simulink model "ROPOD_Control_SIM"  (R2017b)
settings: Solver=VariableStepAuto  StartTime=0.0  StopTime=inf  RelTol=1e-3
values from neighbouring files (symbols this model uses):
  AgentNumber = 1    [init_model.m]
  FFtheta_intia = 0    [init_model.m]
  FFxy_mass = 0*80    (= 0)    [init_model.m]
  flock_FFtheta_friction = 50    [init_model.m]
  flock_FFxy_friction = 100    [init_model.m]
  I_fhz_ddelta_cntr = 0    [init_model.m]
  I_fhz_dtheta_cntr = 0.3    [init_model.m]
  I_fhz_dtheta_flock_cntr = 0.1    [init_model.m]
  I_fhz_dvarphi_cntr = 0    [init_model.m]
  I_fhz_dxdy_cntr = 0.25    [init_model.m]
  I_fhz_dxdy_flock_cntr = 0.1    [init_model.m]
  K_gain_ddelta_cntr = 0.1    [init_model.m]
  K_gain_dtheta_cntr = 150    [init_model.m]
  K_gain_dtheta_flock_cntr = 100    [init_model.m]
  K_gain_dvarphi_cntr = 0.05    [init_model.m]
  K_gain_dxdy_cntr = 200    [init_model.m]
  K_gain_dxdy_flock_cntr = 200    [init_model.m]
  LL_wp_fhz_ddelta_cntr = 2    [init_model.m]
  LL_wp_fhz_dtheta_cntr = 20    [init_model.m]
  LL_wp_fhz_dtheta_flock_cntr = 20    [init_model.m]
  LL_wp_fhz_dvarphi_cntr = 10    [init_model.m]
  LL_wp_fhz_dxdy_cntr = 20    [init_model.m]
  LL_wp_fhz_dxdy_flock_cntr = 20    [init_model.m]
  LL_wz_fhz_ddelta_cntr = 2    [init_model.m]
  LL_wz_fhz_dtheta_cntr = 20    [init_model.m]
  LL_wz_fhz_dtheta_flock_cntr = 20    [init_model.m]
  LL_wz_fhz_dvarphi_cntr = 2    [init_model.m]
  LL_wz_fhz_dxdy_cntr = 20    [init_model.m]
  LL_wz_fhz_dxdy_flock_cntr = 20    [init_model.m]
  LPF_fhz_ddelta_cntr = 50    [init_model.m]
  LPF_fhz_ddelta_meas = 50    [init_model.m]
  LPF_fhz_dtheta_cntr = 100    [init_model.m]
  LPF_fhz_dtheta_flock_cntr = 40    [init_model.m]
  LPF_fhz_dvarphi_cntr = 50    [init_model.m]
  LPF_fhz_dvarphi_meas = 50    [init_model.m]
  LPF_fhz_dxdy_cntr = 100    [init_model.m]
  LPF_fhz_dxdy_flock_cntr = 40    [init_model.m]
  max_flock_acc_theta = 0.5    [init_model.m]
  max_flock_acc_xy = 0.5    [init_model.m]
  max_flock_vel_theta = 1.0    (= 1)    [init_model.m]
  max_flock_vel_xy = 1.0    (= 1)    [init_model.m]
  max_hw_tau = 7.0    (= 7)    [init_model.m]
  max_ropod_acc_theta = 1.6    [init_model.m]
  max_ropod_acc_xy = 2.0    (= 2)    [init_model.m]
  max_ropod_sw_force = 500    [init_model.m]
  max_ropod_sw_tau = 250    [init_model.m]
  max_ropod_vel_theta = 1.6    [init_model.m]
  max_ropod_vel_xy = 2.0    (= 2)    [init_model.m]
  max_sw_current = 10    [init_model.m]
  Nagents = 2    [init_model.m]
  Nwheels = 4    [Jqwl_numeric_function.m]    (also in S_matrix.m; extract_kinmodel_parameters.m; init_model.m; tau_optimal_dist_vec_fun.m)
  pivot_offs_sws = [0.0243    0.4689    0.3384    5.9050]    [init_model.m]
  ropod_kinmodel_pv = struct2array(ropod_kinmodel_param)    [set_ropod_KinModparams.m]
  ropod_position_inflock = [-1 0 3.1416]    [init_model.m]
  SW_COM1_ENABLE1 = hex2dec('0001')    [init_model.m]
  SW_COM1_ENABLE2 = hex2dec('0002')    [init_model.m]
  SW_COM1_MODE_TORQUE = bitshift(hex2dec('0000'),2)    [init_model.m]
  SW_COM1_MODE_VELOCITY = bitshift(hex2dec('0002'),2)    [init_model.m]
  SW_COM1_USE_TS = hex2dec('8000')    [init_model.m]
  sw_tau_2_current = 1/motor_physical_parameters.torqueconstant.value    [init_model.m]
  Tinit = 2    [init_model.m]
  Ts = 0.001    [init_model.m]
  Ts_MPC = 0.01    [init_model.m]
  Tsflck = 0.01    [init_model.m]
undefined symbols (not defined in the file or in its folder): acc_limit, accmax, b_cx, b_cy, b_rx, bus_size, comp_enable, Desired, DiscIntNeverNeededParam, Fcgain, gdis, k_cx, k_cy, live_tuning, m_robot, Nominal, Nominal_x, Nominal_y, offsets, portwidth, sizes, types, vel_limit, vmax1, vmax2
libraries: simulink x90, cstblocks x66, dspsigops x12, dspnetwork x4
(part 3 of 8)

== system ROPOD_Control_SIM/RopodTorqueDistribution/wheel flip compensation ==
  varphi_tau_sp_in : Inport
  ropod_kin_param : Inport  Port=2
  flip_comp_factor : Inport  Port=3
  sw_conf : Inport  Port=4
  Bus Selector1 : BusSelector  OutputSignals=max_current,sw_tau_2_current
  Constant : Constant  Value=10
  Demux : Demux  Outputs=8
  Divide : Product  Inputs=*/
  MATLAB Function1 : MATLAB Function  TreatAsAtomicUnit=on
  MATLAB Function2 : MATLAB Function  TreatAsAtomicUnit=on
  MATLAB Function3 : MATLAB Function  TreatAsAtomicUnit=on
  MATLAB Function4 : MATLAB Function  TreatAsAtomicUnit=on
  Mux : Mux  Inputs=8
  Terminator{,1..3} (4 alike) : Terminator
  varphi_tau_sp_out : Outport
  wires:
  varphi_tau_sp_in/1 -> Demux/1
  ropod_kin_param/1 -> [ropod_kin_param]
  flip_comp_factor/1 -> [kmax]
  Demux/2 -> MATLAB Function4/2(tr)
  Demux/1 -> MATLAB Function4/1(tl)
  [kmax] -> MATLAB Function4/4(kmax)
  [ropod_kin_param] -> MATLAB Function4/3(ropod_kinmodel_param_vec)
  MATLAB Function4/1(tl_out) -> Mux/1
  MATLAB Function4/2(tr_out) -> Mux/2
  MATLAB Function4/3(sc) -> Terminator/1
  Mux/1 -> varphi_tau_sp_out/1
  Constant/1 -> [Fthr]
  [Fthr] -> MATLAB Function4/5(Fthr)
  Divide/1 -> [tau_max]
  [tau_max] -> MATLAB Function4/6(tau_max)
  MATLAB Function1/3(sc) -> Terminator1/1
  Demux/4 -> MATLAB Function1/2(tr)
  [Fthr] -> MATLAB Function1/5(Fthr)
  MATLAB Function1/2(tr_out) -> Mux/4
  Demux/3 -> MATLAB Function1/1(tl)
  [ropod_kin_param] -> MATLAB Function1/3(ropod_kinmodel_param_vec)
  [kmax] -> MATLAB Function1/4(kmax)
  MATLAB Function1/1(tl_out) -> Mux/3
  [tau_max] -> MATLAB Function1/6(tau_max)
  Demux/7 -> MATLAB Function3/1(tl)
  [kmax] -> MATLAB Function3/4(kmax)
  Demux/8 -> MATLAB Function3/2(tr)
  [ropod_kin_param] -> MATLAB Function2/3(ropod_kinmodel_param_vec)
  MATLAB Function3/2(tr_out) -> Mux/8
  Demux/5 -> MATLAB Function2/1(tl)
  [tau_max] -> MATLAB Function2/6(tau_max)
  [tau_max] -> MATLAB Function3/6(tau_max)
  [Fthr] -> MATLAB Function2/5(Fthr)
  MATLAB Function3/1(tl_out) -> Mux/7
  [Fthr] -> MATLAB Function3/5(Fthr)
  MATLAB Function2/3(sc) -> Terminator2/1
  MATLAB Function3/3(sc) -> Terminator3/1
  MATLAB Function2/2(tr_out) -> Mux/6
  [kmax] -> MATLAB Function2/4(kmax)
  Demux/6 -> MATLAB Function2/2(tr)
  [ropod_kin_param] -> MATLAB Function3/3(ropod_kinmodel_param_vec)
  MATLAB Function2/1(tl_out) -> Mux/5
  Bus Selector1/1 -> Divide/1  "<max_current>"
  Bus Selector1/2 -> Divide/2  "<sw_tau_2_current>"
  sw_conf/1 -> Bus Selector1/1

== system ROPOD_Control_SIM/RopodTorqueDistribution/wheel vel cntr ==
  platform_dxdy_cntr_param : Inport
  disable : Inport  Port=2
  dvarphi_sp : Inport  Port=3
  ena_w : Inport  Port=4
  dvarphi : Inport  Port=5
  Sum : Sum  Inputs=-+|
  Wheels Velocity controller : Subsystem
  varphi_tau_setp_out : Outport
  wires:
  Wheels Velocity controller/1(varphi_tau_setp) -> varphi_tau_setp_out/1
  ena_w/1 -> Wheels Velocity controller/2(ena_w)
  Sum/1 -> Wheels Velocity controller/1(dvarphi_error)
  dvarphi/1 -> Sum/1
  dvarphi_sp/1 -> Sum/2
  disable/1 -> Wheels Velocity controller/4(reset_int)
  platform_dxdy_cntr_param/1 -> Wheels Velocity controller/3(platform_dvarphi_cntr_param)

== system ROPOD_Control_SIM/RopodVelocityController/Platorm Velocity controller ==
  note: Mass Feedforward
  reset_int : Inport
  platform_dxdy_cntr_param : Inport  Port=2
  platform_dtheta_cntr_param : Inport  Port=3
  dqr_sp : Inport  Port=4
  dqr_loc : Inport  Port=5
  Demux : Demux  Outputs=3
  Demux1 : Demux  Outputs=3
  Discrete Derivative : simulink/Discrete/Discrete Derivative  gainval=1.0  ICPrevScaledInput=0.0  OutMin=[]  OutMax=[]  OutDataType=fixdt(1, 16)  OutScaling=2^-10  DoSatur=off
  G_I_LL_LPF Controller_X : Subsystem
  G_I_LL_LPF Controller_Y : Subsystem
  G_I_LL_LPF Controller_theta : Subsystem
  Gain : Gain  Gain=FFxy_mass
  Gain1 : Gain  Gain=FFxy_mass
  Gain2 : Gain  Gain=FFtheta_intia
  Mux : Mux  Inputs=3
  Mux1 : Mux  Inputs=3
  Signal Specification : SignalSpecification  Dimensions=3
  Sum : Sum  Inputs=|+-
  Sum1 : Sum  Inputs=++|
  w_platform_setp : Outport
  wires:
  Sum/1 -> Demux/1
  G_I_LL_LPF Controller_theta/1(Out) -> Mux/3
  Demux/1 -> G_I_LL_LPF Controller_X/2(In)
  Demux/2 -> G_I_LL_LPF Controller_Y/2(In)
  G_I_LL_LPF Controller_Y/1(Out) -> Mux/2
  G_I_LL_LPF Controller_X/1(Out) -> Mux/1
  Demux/3 -> G_I_LL_LPF Controller_theta/2(In)
  dqr_sp/1 -> Sum/1, Discrete Derivative/1
  dqr_loc/1 -> Sum/2
  [param_dxdy_cntr] -> G_I_LL_LPF Controller_X/1(param)
  [param_dxdy_cntr] -> G_I_LL_LPF Controller_Y/1(param)
  [param_dtheta_cntr] -> G_I_LL_LPF Controller_theta/1(param)
  reset_int/1 -> [reset_int_cntr]
  [reset_int_cntr] -> G_I_LL_LPF Controller_X/3(reset_integrator)
  [reset_int_cntr] -> G_I_LL_LPF Controller_Y/3(reset_integrator)
  platform_dxdy_cntr_param/1 -> [param_dxdy_cntr]
  platform_dtheta_cntr_param/1 -> [param_dtheta_cntr]
  [reset_int_cntr] -> G_I_LL_LPF Controller_theta/3(reset_integrator)
  Discrete Derivative/1 -> Demux1/1
  Demux1/1 -> Gain/1
  Gain/1 -> Mux1/1
  Demux1/2 -> Gain1/1
  Gain1/1 -> Mux1/2
  Demux1/3 -> Gain2/1
  Gain2/1 -> Mux1/3
  Sum1/1 -> Signal Specification/1
  Mux1/1 -> Sum1/1
  Mux/1 -> Sum1/2
  Signal Specification/1 -> w_platform_setp/1

== system ROPOD_Control_SIM/RopodVelocityController/Subscriber vel commands1 ==
  note: set 0 for testing
  note: if no vel commands are received after 0.5 sec, stop
  base_conf : Inport
  new_cmd : Inport  Port=2
  dq_setp : Inport  Port=3
  Bus Selector1 : BusSelector  OutputSignals=max_acc_xy,max_vel_xy
  Bus Selector2 : BusSelector  OutputSignals=max_acc_xy,max_vel_xy
  Bus Selector3 : BusSelector  OutputSignals=max_acc_theta,max_vel_theta
  Compare To Constant : simulink/Logic and Bit Operations/Compare To Constant  relop=>=  const=0.5  OutDataTypeStr=boolean
  Constant : Constant  Value=0  SampleTime=Ts
  Constant1 : Constant  Value=0
  Constant2 : Constant  Value=0
  Demux : Demux  Outputs=3
  Digital Clock : DigitalClock  SampleTime=Ts
  Enabled Delay : Delay  DelayLength=1  ShowEnablePort=on  SampleTime=Ts
      settings: InputPortMap=u0,e6
  Gain{,1..5} (6 alike) : Gain  Gain=-1
  Gain6 : Gain
  Mux : Mux  Inputs=3
  Rate Limiter Dynamic : simulink/Discontinuities/Rate Limiter Dynamic
      settings: SourceProductName=Simulink
  Rate Limiter Dynamic1 : simulink/Discontinuities/Rate Limiter Dynamic
      settings: SourceProductName=Simulink
  Rate Limiter Dynamic2 : simulink/Discontinuities/Rate Limiter Dynamic
      settings: SourceProductName=Simulink
  Saturation Dynamic : simulink/Discontinuities/Saturation Dynamic  OutMin=[]  OutMax=[]  OutDataTypeStr=Inherit: Same as second input  OutDataType=fixdt(1, 16)  OutScaling=2^-10  DoSatur=off
  Saturation Dynamic1 : simulink/Discontinuities/Saturation Dynamic  OutMin=[]  OutMax=[]  OutDataTypeStr=Inherit: Same as second input  OutDataType=fixdt(1, 16)  OutScaling=2^-10  DoSatur=off
  Saturation Dynamic2 : simulink/Discontinuities/Saturation Dynamic  OutMin=[]  OutMax=[]  OutDataTypeStr=Inherit: Same as second input  OutDataType=fixdt(1, 16)  OutScaling=2^-10  DoSatur=off
  Subtract : Sum  Inputs=+-
  Switch : Switch  Criteria=u2 > Threshold
  Switch1 : Switch  Criteria=u2 > Threshold
  Switch2 : Switch  Criteria=u2 > Threshold
  dq_loc_sp : Outport
  wires:
  Demux/1 -> Switch/3
  dq_setp/1 -> Demux/1
  new_cmd/1 -> Enabled Delay/2
  Digital Clock/1 -> Enabled Delay/1, Subtract/1
  Enabled Delay/1 -> Subtract/2
  Subtract/1 -> Compare To Constant/1
  Constant/1 -> Switch/1
  Gain/1 -> Rate Limiter Dynamic/3
  Switch/1 -> Saturation Dynamic/2
  Gain1/1 -> Saturation Dynamic/3
  Saturation Dynamic/1 -> Rate Limiter Dynamic/2
  Switch1/1 -> Saturation Dynamic1/2
  Gain3/1 -> Saturation Dynamic1/3
  Constant1/1 -> Switch1/1
  Demux/2 -> Switch1/3
  Gain2/1 -> Rate Limiter Dynamic1/3
  Saturation Dynamic1/1 -> Rate Limiter Dynamic1/2
  Bus Selector2/1 -> Rate Limiter Dynamic1/1, Gain2/1  "<max_acc_xy>"
  Bus Selector2/2 -> Saturation Dynamic1/1, Gain3/1  "<max_vel_xy>"
  Bus Selector3/1 -> Rate Limiter Dynamic2/1, Gain4/1  "<max_acc_theta>"
  Saturation Dynamic2/1 -> Rate Limiter Dynamic2/2
  base_conf/1 -> Bus Selector3/1, Bus Selector2/1, Bus Selector1/1
  Switch2/1 -> Saturation Dynamic2/2
  Constant2/1 -> Switch2/1
  Demux/3 -> Switch2/3
  Gain5/1 -> Saturation Dynamic2/3
  Gain4/1 -> Rate Limiter Dynamic2/3
  Compare To Constant/1 -> Gain6/1
  Bus Selector3/2 -> Saturation Dynamic2/1, Gain5/1  "<max_vel_theta>"
  Mux/1 -> dq_loc_sp/1
  Rate Limiter Dynamic/1 -> Mux/1
  Rate Limiter Dynamic1/1 -> Mux/2
  Rate Limiter Dynamic2/1 -> Mux/3
  Bus Selector1/2 -> Saturation Dynamic/1, Gain1/1  "<max_vel_xy>"
  Bus Selector1/1 -> Rate Limiter Dynamic/1, Gain/1  "<max_acc_xy>"
  Gain6/1 -> Switch2/2, Switch1/2, Switch/2

== system ROPOD_Control_SIM/Subsystem/Ropod kinematic parameters ==
  ropod_kinmodel_pv : Constant  Value=ropod_kinmodel_pv
  ropod_kin_param : Outport
  wires:
  ropod_kinmodel_pv/1 -> ropod_kin_param/1

== system ROPOD_Control_SIM/Subsystem/Smart wheels conf1 ==
  Bus Creator : BusCreator  Inputs=9
  LPF_fhz_ddelta_meas : Constant  Value=LPF_fhz_ddelta_meas
  LPF_fhz_dvarphi_meas : Constant  Value=LPF_fhz_dvarphi_meas
  enable : Constant
  max_current : Constant  Value=max_sw_current
  pivot_offset_sw1 : Constant  Value=pivot_offs_sws(1)
  pivot_offset_sw2 : Constant  Value=pivot_offs_sws(2)
  pivot_offset_sw3 : Constant  Value=pivot_offs_sws(3)
  pivot_offset_sw4 : Constant  Value=pivot_offs_sws(4)
  sw_tau_2_current : Constant  Value=sw_tau_2_current
  sw_conf : Outport
  wires:
  enable/1 -> Bus Creator/1  "enable"
  max_current/1 -> Bus Creator/2  "max_current"
  pivot_offset_sw1/1 -> Bus Creator/4  "pivot_offs_sw1"
  pivot_offset_sw2/1 -> Bus Creator/5  "pivot_offs_sw2"
  pivot_offset_sw3/1 -> Bus Creator/6  "pivot_offs_sw3"
  pivot_offset_sw4/1 -> Bus Creator/7  "pivot_offs_sw4"
  LPF_fhz_dvarphi_meas/1 -> Bus Creator/8  "dvarphi_LPF_fhz"
  LPF_fhz_ddelta_meas/1 -> Bus Creator/9  "ddelta_LPF_fhz"
  Bus Creator/1 -> sw_conf/1
  sw_tau_2_current/1 -> Bus Creator/3  "sw_tau_2_current"

== system ROPOD_Control_SIM/Subsystem1/Compliant control ==
  Forces : Inport
  states : Inport  Port=2
  motion tuning bus : Inport  Port=3
  Demux : Demux  Outputs=3
  Gain : Gain  Gain=comp_enable
  Gain4 : Gain  Gain=Fcgain
  Ground [3,1] : Subsystem
  Ground [3,1]1 : Subsystem
  Ground [3,1]2 : Subsystem
  Impedance : Subsystem
  Manual Switch : ManualSwitch  CurrentSetting=0
  Force_out : Outport
  wires:
  Manual Switch/1 -> Gain/1
  Forces/1 -> Impedance/7(Fext), Gain4/1
  Impedance/1(Imp_force) -> Manual Switch/2
  Gain4/1 -> Manual Switch/1
  states/1 -> Demux/1
  Demux/2 -> Impedance/5(y)
  Demux/1 -> Impedance/4(x)
  Demux/3 -> Impedance/6(theta)
  Gain/1 -> Force_out/1
  motion tuning bus/1 -> Impedance/8(motion tuning bus)
  Ground [3,1]/1(Out1) -> Impedance/1(X0)
  Ground [3,1]1/1(Out1) -> Impedance/2(Y0)
  Ground [3,1]2/1(Out1) -> Impedance/3(theta0i)

== system ROPOD_Control_SIM/Subsystem1/Observer ==
  Input_force : Inport
  states : Inport  Port=2
  DOB3 : Subsystem
  DOB_x : Subsystem  Commented=on
  DOB_y : Subsystem  Commented=on
  Demux1 : Demux  Outputs=3
  To Workspace2 : ToWorkspace  VariableName=est_dist  SampleTime=-1
  Force_obs : Outport
  wires:
  Input_force/1 -> DOB3/1(Control input)
  DOB3/1(Estimated disturbance) -> Force_obs/1, To Workspace2/1
  states/1 -> Demux1/1
  Demux1/1 -> DOB3/2(x)
  Demux1/2 -> DOB3/3(y)
  Demux1/3 -> DOB3/4(theta)

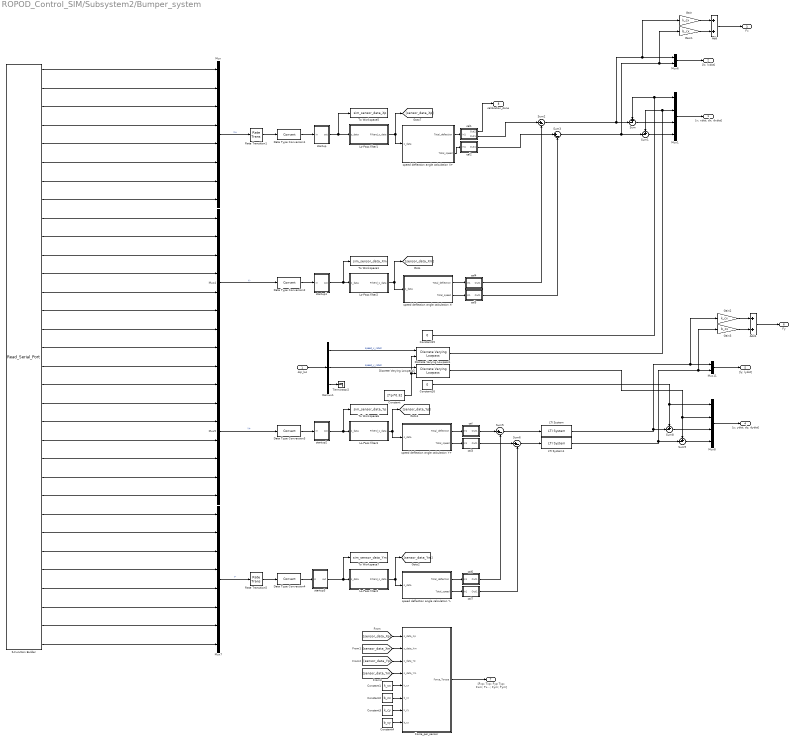
== system ROPOD_Control_SIM/Subsystem2/Bumper_system ==
  dqr_loc : Inport
  Add : Sum
  Add1 : Sum
  Constant : Constant  Value=2*pi*0.32
  Constant1 : Constant  Value=k_cx
  Constant15 : Constant  Value=0
  Constant16 : Constant  Value=0
  Constant2 : Constant  Value=b_cx
  Constant3 : Constant  Value=k_cy
  Constant4 : Constant  Value=b_cy
  Data Type Conversion{1..4} (4 alike) : DataTypeConversion
  Demux1 : Demux  Outputs=3
  Discrete Varying Lowpass1 : cstblocks/Linear Parameter Varying/Discrete Varying Lowpass  N=1  w0=0  Ts=Ts_MPC
      settings: SourceProductName=Control System Toolbox  SourceProductBaseCode=CT
  Discrete Varying Lowpass3 : cstblocks/Linear Parameter Varying/Discrete Varying Lowpass  N=1  w0=0  Ts=Ts_MPC
      settings: SourceProductName=Control System Toolbox  SourceProductBaseCode=CT
  Force_per_sensor : MATLAB Function  TreatAsAtomicUnit=on
  Gain : Gain  Gain=k_cx
  Gain1 : Gain  Gain=b_cx
  Gain2 : Gain  Gain=k_cx
  Gain3 : Gain  Gain=b_cx
  LTI System : cstblocks/LTI System  sys=hpfD_Bumper  IC=[]
  LTI System1 : cstblocks/LTI System  sys=hpfD_Bumper  IC=[]
  Lo-Pass filter1 : Subsystem
  Lo-Pass filter2 : Subsystem
  Lo-Pass filter3 : Subsystem
  Lo-Pass filter4 : Subsystem
  Mux{,4..5,7} (4 alike) : Mux  Inputs=8
  Mux1 : Mux
  Mux11 : Mux  Inputs=2
  Mux6 : Mux  Inputs=2
  Mux8 : Mux
  Rate Transition1 : RateTransition  OutPortSampleTime=Ts_MPC
  Rate Transition5 : RateTransition  OutPortSampleTime=Ts_MPC
  S-Function Builder : S-Function  InitFcn=try, set_param(gcb,'FunctionName','Read_Serial_Port'), end  FunctionName=Read_Serial_Port  SFunctionModules=Read_Serial_Port_wrapper  SFunctionDeploymentMode=off  EnableBusSupport=off  mask(S-Function Builder){}
      mask help: Simulink:masks:SFunctionBuilder_MD
      mask init:
      | val = [[.9  0.75 0.75 1 1 .9 .9 1]',[1 1 0.75 0.75 .9 .9 1 .9]'];try , sys = get_param(gcb,'SfunBuilderFcnName');if isempty(sys), sys = get_param(gcb,'FunctionName'); end,catch, sys = get_param(gcb,'FunctionName'); end
      settings: CopyFcn=set_param(gcbh,'LinkStatus','none')  PreSaveFcn=try, set_param(gcb,'FunctionName','Read_Serial_Port'), end  OpenFcn=sfunctionwizard(gcbh)
      mask Display: plot(val(:,1),val(:,2)),disp(sys), port_label('output',1,'dxp1'), port_label('output',2,'dxp2'), port_label('output',3,'dxp3'), port_label('output',4,'dxp4'), port_label('output',5,'sxp1'), port_label('output',6,'sxp2'), port_label('output',7,'sxp3'), port_label('output',8,'sxp4'), port_label('output',9,'dxm1'), port_label('output',10,'dxm2'), port_label('output',11,'dxm3'), port_label('output',12,'dxm4'), port_label('output',13,'sxm1'), port_label('output',14,'sxm2'), port_label('output',15,'sxm3'), port_label('output',16,'sxm4'), port_label('output',17,'dyp1'), port_label('output',18,'dyp2'), port_label('output',19,'dyp3'), port_label('output',20,'dyp4'), port_label('output',21,'syp1'), port_label('output',22,'syp2'), port_label('output',23,'syp3'), port_label('output',24,'syp4'), port_label('output',25,'dym1'), port_label('output',26,'dym2'), port_label('output',27,'dym3'), port_label('output',28,'dym4'), port_label('output',29,'sym1'), port_label('output',30,'sym2'), port_label('output',31,'sym3'), port_label('output',32,'sym4')
  Sum{,1,8..9} (4 alike) : Sum  Inputs=+-|
  Sum{2..3,5..6} (4 alike) : Sum  Inputs=|+-
  Terminator2 : Terminator
  To Workspace1 : ToWorkspace  VariableName=sim_sensor_data_Xm  SampleTime=-1
      settings: Save2DSignal=2-D array (concatenate along first dimension)
  To Workspace5 : ToWorkspace  VariableName=sim_sensor_data_Xp  SampleTime=-1
      settings: Save2DSignal=2-D array (concatenate along first dimension)
  To Workspace6 : ToWorkspace  VariableName=sim_sensor_data_Yp  SampleTime=-1
      settings: Save2DSignal=2-D array (concatenate along first dimension)
  To Workspace7 : ToWorkspace  VariableName=sim_sensor_data_Ym  SampleTime=-1
      settings: Save2DSignal=2-D array (concatenate along first dimension)
  cal : Subsystem
  cal1 : Subsystem
  cal2 : Subsystem
  cal3 : Subsystem
  cal4 : Subsystem
  cal5 : Subsystem
  cal6 : Subsystem
  cal7 : Subsystem
  speed deflection angle calculation X+ : MATLAB Function  TreatAsAtomicUnit=on
  speed deflection angle calculation X- : MATLAB Function  TreatAsAtomicUnit=on
  speed deflection angle calculation Y+ : MATLAB Function  TreatAsAtomicUnit=on
  speed deflection angle calculation Y- : MATLAB Function  TreatAsAtomicUnit=on
  startup : Subsystem
  startup1 : Subsystem
  startup2 : Subsystem
  startup3 : Subsystem
  "[x; xdot; dx; dxdot]" : Outport
  "[lx; lxdot]" : Outport  Port=2
  Fx : Outport  Port=3
  "[y; ydot; dy; dydot]" : Outport  Port=4
  "[ly; lydot]" : Outport  Port=5
  Fy : Outport  Port=6
  "[Fxp; Txp; Fyp Typ; Fxm; Txm; Fym; Tym] " : Outport  Port=7
  calibration_done : Outport  Port=8
  wires:
  Mux6/1 -> "[lx; lxdot]"/1
  Mux1/1 -> "[x; xdot; dx; dxdot]"/1
  Sum/1 -> Mux1/3
  Constant15/1 -> Mux1/1, Sum/1
  Sum1/1 -> Mux1/4
  Demux1/3 -> Terminator2/1
  Demux1/1 -> Discrete Varying Lowpass1/1  "speed_x_robot"
  dqr_loc/1 -> Demux1/1
  Demux1/2 -> Discrete Varying Lowpass3/1  "speed_y_robot"
  Mux/1 -> Rate Transition1/1  "X+"
  Lo-Pass filter1/1(Filterd_s_data) -> [sensor_data_Xp], speed deflection angle calculation X+/1(s_data)
  Data Type Conversion1/1 -> startup/1(in)
  Rate Transition1/1 -> Data Type Conversion1/1
  Data Type Conversion2/1 -> startup1/1(in)
  Mux4/1 -> Data Type Conversion2/1  "X-"
  Data Type Conversion3/1 -> startup2/1(in)
  Lo-Pass filter3/1(Filterd_s_data) -> speed deflection angle calculation Y+/1(s_data), [sensor_data_Yp]
  Rate Transition5/1 -> Data Type Conversion4/1
  Data Type Conversion4/1 -> startup3/1(in)
  Lo-Pass filter4/1(Filterd_s_data) -> speed deflection angle calculation Y-/1(s_data), [sensor_data_Ym]
  Mux7/1 -> Rate Transition5/1  "Y-"
  Mux5/1 -> Data Type Conversion3/1  "Y+"
  speed deflection angle calculation X+/1(Total_deflection) -> cal1/1(In1)
  cal4/1(Out1) -> Sum2/2
  cal5/1(Out1) -> Sum3/2
  speed deflection angle calculation Y-/1(Total_deflection) -> cal6/1(In1)
  speed deflection angle calculation Y+/2(Total_speed) -> cal3/1(In1)
  speed deflection angle calculation Y-/2(Total_speed) -> cal7/1(In1)
  Sum8/1 -> Mux8/3
  Mux8/1 -> "[y; ydot; dy; dydot]"/1
  Constant16/1 -> Mux8/1, Sum8/1
  Mux11/1 -> "[ly; lydot]"/1
  Sum9/1 -> Mux8/4
  Discrete Varying Lowpass3/1 -> Mux8/2, Sum9/1
  Sum5/1 -> LTI System/1
  Sum2/1 -> Sum/2, Gain/1, Mux6/1
  Sum3/1 -> Sum1/2, Gain1/1, Mux6/2
  Sum6/1 -> LTI System1/1
  startup/1(out) -> To Workspace5/1, Lo-Pass filter1/1(s_data)
  startup1/1(out) -> Lo-Pass filter2/1(s_data), To Workspace1/1
  startup2/1(out) -> Lo-Pass filter3/1(s_data), To Workspace6/1
  startup3/1(out) -> Lo-Pass filter4/1(s_data), To Workspace7/1
  Constant/1 -> Discrete Varying Lowpass3/2, Discrete Varying Lowpass1/2
  S-Function Builder/26 -> Mux7/2
  S-Function Builder/31 -> Mux7/7
  S-Function Builder/20 -> Mux5/4
  S-Function Builder/18 -> Mux5/2
  S-Function Builder/25 -> Mux7/1
  S-Function Builder/13 -> Mux4/5
  S-Function Builder/23 -> Mux5/7
  S-Function Builder/15 -> Mux4/7
  S-Function Builder/22 -> Mux5/6
  S-Function Builder/14 -> Mux4/6
  S-Function Builder/17 -> Mux5/1
  S-Function Builder/32 -> Mux7/8
  S-Function Builder/7 -> Mux/7
  S-Function Builder/19 -> Mux5/3
  S-Function Builder/21 -> Mux5/5
  S-Function Builder/8 -> Mux/8
  S-Function Builder/5 -> Mux/5
  S-Function Builder/4 -> Mux/4
  S-Function Builder/29 -> Mux7/5
  S-Function Builder/6 -> Mux/6
  S-Function Builder/1 -> Mux/1
  S-Function Builder/3 -> Mux/3
  S-Function Builder/10 -> Mux4/2
  S-Function Builder/11 -> Mux4/3
  S-Function Builder/12 -> Mux4/4
  S-Function Builder/16 -> Mux4/8
  S-Function Builder/28 -> Mux7/4
  S-Function Builder/27 -> Mux7/3
  S-Function Builder/9 -> Mux4/1
  S-Function Builder/30 -> Mux7/6
  S-Function Builder/2 -> Mux/2
  S-Function Builder/24 -> Mux5/8
  [sensor_data_Xp] -> Force_per_sensor/1(s_data_Xp)
  [sensor_data_Xm] -> Force_per_sensor/2(s_data_Xm)
  [sensor_data_Yp] -> Force_per_sensor/3(s_data_Yp)
  [sensor_data_Ym] -> Force_per_sensor/4(s_data_Ym)
  Force_per_sensor/1(Force_Torque) -> "[Fxp; Txp; Fyp Typ; Fxm; Txm; Fym; Tym] "/1
  Constant1/1 -> Force_per_sensor/5(k_cx)
  Constant2/1 -> Force_per_sensor/6(b_cx)
  Constant3/1 -> Force_per_sensor/7(k_cy)
  Constant4/1 -> Force_per_sensor/8(b_cy)
  speed deflection angle calculation X+/2(Total_speed) -> cal2/1(In1)
  speed deflection angle calculation X-/1(Total_deflection) -> cal4/1(In1)
  speed deflection angle calculation X-/2(Total_speed) -> cal5/1(In1)
  speed deflection angle calculation Y+/1(Total_deflection) -> cal/1(In1)
  cal/1(Out1) -> Sum5/1
  cal3/1(Out1) -> Sum6/1
  cal6/1(Out1) -> Sum5/2
  cal7/1(Out1) -> Sum6/2
  cal1/2(Out1) -> Sum2/1
  cal2/1(Out1) -> Sum3/1
  Lo-Pass filter2/1(Filterd_s_data) -> speed deflection angle calculation X-/1(s_data), [sensor_data_Xm]
  Discrete Varying Lowpass1/1 -> Sum1/1, Mux1/2
  cal1/1(Out2) -> calibration_done/1
  Gain/1 -> Add/1
  Gain1/1 -> Add/2
  Add/1 -> Fx/1
  Gain2/1 -> Add1/1
  LTI System1/1 -> Sum9/2, Gain3/1, Mux11/2
  Add1/1 -> Fy/1
  LTI System/1 -> Sum8/2, Gain2/1, Mux11/1
  Gain3/1 -> Add1/2

== system ROPOD_Control_SIM/Subsystem2/ZMPC_1d_x ==
  update_parameters : Inport
  "[x; xdot; d; ddot]" : Inport  Port=2
  Fd_max : Inport  Port=3
  Fd_min : Inport  Port=4
  l_max : Inport  Port=5
  l_min : Inport  Port=6
  Fr_max : Inport  Port=7
  Fr_min : Inport  Port=8
  m_r : Inport  Port=9
  b_r : Inport  Port=10
  b_c : Inport  Port=11
  k_c : Inport  Port=12
  Ts_MPC : Inport  Port=13
  Enable : EnablePort  StatesWhenEnabling=reset
  MATLAB Function : MATLAB Function  TreatAsAtomicUnit=on
  Zone MPC : MATLAB Function  TreatAsAtomicUnit=on  SystemSampleTime=Ts_MPC
  epsilon : Outport  OutputWhenDisabled=reset  InitialOutput=0
  Fx : Outport  Port=2  OutputWhenDisabled=reset  InitialOutput=0
  Feasability : Outport  Port=3  OutputWhenDisabled=reset  InitialOutput=0
  wires:
  Zone MPC/3(exitflag) -> Feasability/1
  "[x; xdot; d; ddot]"/1 -> Zone MPC/1(xk)
  Zone MPC/1(epsilon) -> epsilon/1
  Zone MPC/2(u_mpc) -> Fx/1
  m_r/1 -> MATLAB Function/1(m_r)
  b_r/1 -> MATLAB Function/2(b_r)
  b_c/1 -> MATLAB Function/3(b_c)
  k_c/1 -> MATLAB Function/4(k_c)
  Fd_max/1 -> MATLAB Function/5(Fd_max)
  Fd_min/1 -> MATLAB Function/6(Fd_min)
  Fr_max/1 -> MATLAB Function/9(Fr_max)
  Fr_min/1 -> MATLAB Function/10(Fr_min)
  Ts_MPC/1 -> MATLAB Function/11(Ts_MPC)
  update_parameters/1 -> MATLAB Function/12(update)
  MATLAB Function/1(F) -> Zone MPC/2(F)
  MATLAB Function/2(W) -> Zone MPC/3(W)
  MATLAB Function/3(c) -> Zone MPC/4(c)
  MATLAB Function/4(H) -> Zone MPC/5(H)
  MATLAB Function/5(A) -> Zone MPC/6(A)
  MATLAB Function/6(rho) -> Zone MPC/7(rho)
  l_max/1 -> MATLAB Function/7(l_max)
  l_min/1 -> MATLAB Function/8(l_min)

== system ROPOD_Control_SIM/Subsystem2/ZMPC_1d_y ==
  update_parameters : Inport
  "[x; xdot; d; ddot]" : Inport  Port=2
  Fd_max : Inport  Port=3
  Fd_min : Inport  Port=4
  l_max : Inport  Port=5
  l_min : Inport  Port=6
  Fr_max : Inport  Port=7
  Fr_min : Inport  Port=8
  m_r : Inport  Port=9
  b_r : Inport  Port=10
  b_c : Inport  Port=11
  k_c : Inport  Port=12
  Ts_MPC : Inport  Port=13
  Enable : EnablePort  StatesWhenEnabling=reset
  MATLAB Function : MATLAB Function  TreatAsAtomicUnit=on
  Zone MPC : MATLAB Function  TreatAsAtomicUnit=on  SystemSampleTime=Ts_MPC
  epsilon : Outport  OutputWhenDisabled=reset  InitialOutput=0
  Fx : Outport  Port=2  OutputWhenDisabled=reset  InitialOutput=0
  Feasability : Outport  Port=3  OutputWhenDisabled=reset  InitialOutput=0
  wires:
  Zone MPC/3(exitflag) -> Feasability/1
  "[x; xdot; d; ddot]"/1 -> Zone MPC/1(xk)
  Zone MPC/1(epsilon) -> epsilon/1
  Zone MPC/2(u_mpc) -> Fx/1
  m_r/1 -> MATLAB Function/1(m_r)
  b_r/1 -> MATLAB Function/2(b_r)
  b_c/1 -> MATLAB Function/3(b_c)
  k_c/1 -> MATLAB Function/4(k_c)
  Fd_max/1 -> MATLAB Function/5(Fd_max)
  Fd_min/1 -> MATLAB Function/6(Fd_min)
  Fr_max/1 -> MATLAB Function/9(Fr_max)
  Fr_min/1 -> MATLAB Function/10(Fr_min)
  Ts_MPC/1 -> MATLAB Function/11(Ts_MPC)
  update_parameters/1 -> MATLAB Function/12(update)
  MATLAB Function/1(F) -> Zone MPC/2(F)
  MATLAB Function/2(W) -> Zone MPC/3(W)
  MATLAB Function/3(c) -> Zone MPC/4(c)
  MATLAB Function/4(H) -> Zone MPC/5(H)
  MATLAB Function/5(A) -> Zone MPC/6(A)
  MATLAB Function/6(rho) -> Zone MPC/7(rho)
  l_max/1 -> MATLAB Function/7(l_max)
  l_min/1 -> MATLAB Function/8(l_min)

== system ROPOD_Control_SIM/FlockController/Flock Velocity controller/G_I_LL_LPF Controller_flock_Theta ==
  param : Inport
  In : Inport  Port=2
  reset_integrator : Inport  Port=3
  Bus Selector : BusSelector  OutputSignals=P_gain,I_freq_hz,LL_zero_fhz,LL_pole_fhz,LPF_fhz
  Discrete Varying Lowpass3 : cstblocks/Linear Parameter Varying/Discrete Varying Lowpass  N=1  w0=0  Ts=Tsflck
      settings: SourceProductName=Control System Toolbox  SourceProductBaseCode=CT
  Gain2 : Gain  Gain=2*pi
  Product5 : Product
  Shapeit Integrator (Tustin) : Subsystem
  Shapeit Lead-Lag (Tustin) : Subsystem
  Out : Outport
  wires:
  Gain2/1 -> Discrete Varying Lowpass3/2
  Product5/1 -> Shapeit Integrator (Tustin)/1(In)
  Discrete Varying Lowpass3/1 -> Out/1
  Shapeit Integrator (Tustin)/1(Out) -> Shapeit Lead-Lag (Tustin)/1(In)
  Bus Selector/1 -> Product5/2  "<P_gain>"
  Bus Selector/2 -> Shapeit Integrator (Tustin)/2(I_fhz)  "<I_freq_hz>"
  param/1 -> Bus Selector/1
  Bus Selector/5 -> Gain2/1  "<LPF_fhz>"
  Bus Selector/4 -> Shapeit Lead-Lag (Tustin)/3(fp)  "<LL_pole_fhz>"
  reset_integrator/1 -> Shapeit Integrator (Tustin)/3(reset)
  Bus Selector/3 -> Shapeit Lead-Lag (Tustin)/2(fz)  "<LL_zero_fhz>"
  Shapeit Lead-Lag (Tustin)/1(Out) -> Discrete Varying Lowpass3/1
  In/1 -> Product5/1

== system ROPOD_Control_SIM/FlockController/Flock Velocity controller/G_I_LL_LPF Controller_flock_X ==
  param : Inport
  In : Inport  Port=2
  reset_integrator : Inport  Port=3
  Bus Selector : BusSelector  OutputSignals=P_gain,I_freq_hz,LL_zero_fhz,LL_pole_fhz,LPF_fhz
  Discrete Varying Lowpass3 : cstblocks/Linear Parameter Varying/Discrete Varying Lowpass  N=1  w0=0  Ts=Tsflck
      settings: SourceProductName=Control System Toolbox  SourceProductBaseCode=CT
  Gain2 : Gain  Gain=2*pi
  Product5 : Product
  Shapeit Integrator (Tustin) : Subsystem
  Shapeit Lead-Lag (Tustin) : Subsystem
  Out : Outport
  wires:
  Gain2/1 -> Discrete Varying Lowpass3/2
  Product5/1 -> Shapeit Integrator (Tustin)/1(In)
  Discrete Varying Lowpass3/1 -> Out/1
  Shapeit Integrator (Tustin)/1(Out) -> Shapeit Lead-Lag (Tustin)/1(In)
  Bus Selector/1 -> Product5/2  "<P_gain>"
  Bus Selector/2 -> Shapeit Integrator (Tustin)/2(I_fhz)  "<I_freq_hz>"
  param/1 -> Bus Selector/1
  Bus Selector/5 -> Gain2/1  "<LPF_fhz>"
  Bus Selector/4 -> Shapeit Lead-Lag (Tustin)/3(fp)  "<LL_pole_fhz>"
  reset_integrator/1 -> Shapeit Integrator (Tustin)/3(reset)
  Bus Selector/3 -> Shapeit Lead-Lag (Tustin)/2(fz)  "<LL_zero_fhz>"
  Shapeit Lead-Lag (Tustin)/1(Out) -> Discrete Varying Lowpass3/1
  In/1 -> Product5/1

== system ROPOD_Control_SIM/FlockController/Flock Velocity controller/G_I_LL_LPF Controller_flock_Y ==
  param : Inport
  In : Inport  Port=2
  reset_integrator : Inport  Port=3
  Bus Selector : BusSelector  OutputSignals=P_gain,I_freq_hz,LL_zero_fhz,LL_pole_fhz,LPF_fhz
  Discrete Varying Lowpass3 : cstblocks/Linear Parameter Varying/Discrete Varying Lowpass  N=1  w0=0  Ts=Tsflck
      settings: SourceProductName=Control System Toolbox  SourceProductBaseCode=CT
  Gain2 : Gain  Gain=2*pi
  Product5 : Product
  Shapeit Integrator (Tustin) : Subsystem
  Shapeit Lead-Lag (Tustin) : Subsystem
  Out : Outport
  wires:
  Gain2/1 -> Discrete Varying Lowpass3/2
  Product5/1 -> Shapeit Integrator (Tustin)/1(In)
  Discrete Varying Lowpass3/1 -> Out/1
  Shapeit Integrator (Tustin)/1(Out) -> Shapeit Lead-Lag (Tustin)/1(In)
  Bus Selector/1 -> Product5/2  "<P_gain>"
  Bus Selector/2 -> Shapeit Integrator (Tustin)/2(I_fhz)  "<I_freq_hz>"
  param/1 -> Bus Selector/1
  Bus Selector/5 -> Gain2/1  "<LPF_fhz>"
  Bus Selector/4 -> Shapeit Lead-Lag (Tustin)/3(fp)  "<LL_pole_fhz>"
  reset_integrator/1 -> Shapeit Integrator (Tustin)/3(reset)
  Bus Selector/3 -> Shapeit Lead-Lag (Tustin)/2(fz)  "<LL_zero_fhz>"
  Shapeit Lead-Lag (Tustin)/1(Out) -> Discrete Varying Lowpass3/1
  In/1 -> Product5/1

== system ROPOD_Control_SIM/RopodTorqueDistribution/ROPOD 4SW/Initialization switch ==
  ropod_cntr_mode : Inport
  curr_setp : Inport  Port=2
  Constant1 : Constant  Value=SW_COM1_MODE_TORQUE
  Constant13 : Constant  Value=SW_COM1_MODE_TORQUE
  Constant5 : Constant  Value=SW_COM1_MODE_VELOCITY
  Index Vector : MultiPortSwitch  DataPortOrder=Zero-based contiguous  zeroidx=on
  Index Vector1 : MultiPortSwitch  DataPortOrder=Zero-based contiguous  zeroidx=on
  Movinf around SW axis center : Constant  Value=[2 -2 2 -2 2 -2 2 -2]
  zeros : Constant  Value=[0 0 0 0 0 0 0 0]
  SW_cntr_mode : Outport
  wheel_setp : Outport  Port=2
  wires:
  ropod_cntr_mode/1 -> Index Vector1/1, Index Vector/1
  Constant1/1 -> Index Vector/2
  zeros/1 -> Index Vector1/2
  Index Vector1/1 -> wheel_setp/1
  Index Vector/1 -> SW_cntr_mode/1
  Constant5/1 -> Index Vector/4
  Constant13/1 -> Index Vector/3
  Movinf around SW axis center/1 -> Index Vector1/4
  curr_setp/1 -> Index Vector1/3

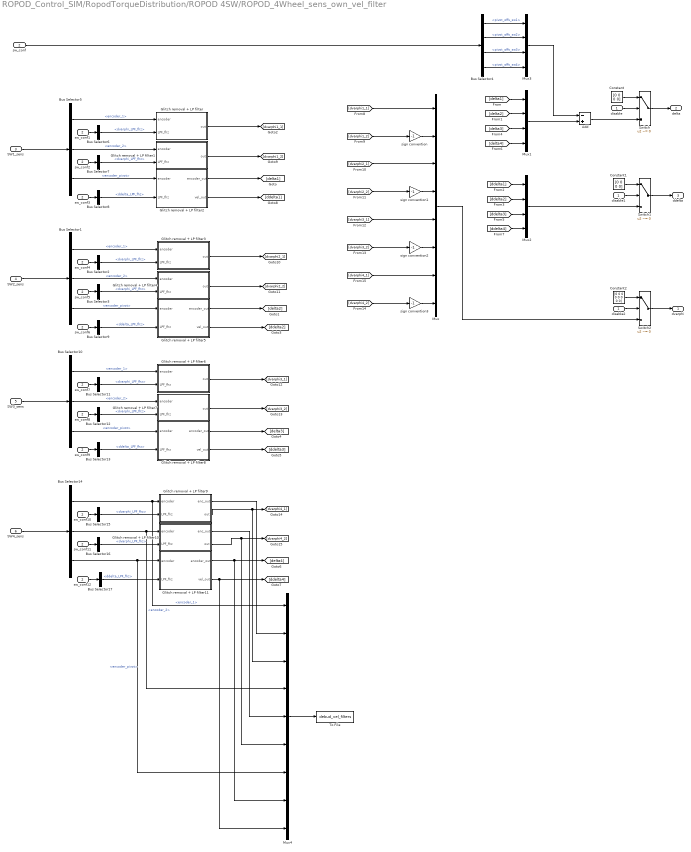
== system ROPOD_Control_SIM/RopodTorqueDistribution/ROPOD 4SW/ROPOD_4Wheel_sens_own_vel_filter ==
  disable : Inport
  sw_conf : Inport  Port=2
  SW1_sens : Inport  Port=3
  SW2_sens : Inport  Port=4
  SW3_sens : Inport  Port=5
  SW4_sens : Inport  Port=6
  Add : Sum  Inputs=-+
  Bus Selector{1,5,10,14} (4 alike) : BusSelector  OutputSignals=encoder_1,encoder_2,encoder_pivot
  Bus Selector{2..3,6..7,11..12,15..16} (8 alike) : BusSelector  OutputSignals=dvarphi_LPF_fhz
  Bus Selector{8..9,13,17} (4 alike) : BusSelector  OutputSignals=ddelta_LPF_fhz
  Bus Selector4 : BusSelector  OutputSignals=pivot_offs_sw1,pivot_offs_sw2,pivot_offs_sw3,pivot_offs_sw4
  Constant : Constant  Value=[0 0 0 0]
  Constant1 : Constant  Value=[0 0 0 0]
  Constant2 : Constant  Value=[0 0 0 0 0 0 0 0]
  Glitch removal + LP filter : Subsystem
  Glitch removal + LP filter1 : Subsystem
  Glitch removal + LP filter10 : Subsystem
  Glitch removal + LP filter11 : Subsystem
  Glitch removal + LP filter2 : Subsystem
  Glitch removal + LP filter3 : Subsystem
  Glitch removal + LP filter4 : Subsystem
  Glitch removal + LP filter5 : Subsystem
  Glitch removal + LP filter6 : Subsystem
  Glitch removal + LP filter7 : Subsystem
  Glitch removal + LP filter8 : Subsystem
  Glitch removal + LP filter9 : Subsystem
  Mux : Mux  Inputs=8
  Mux1 : Mux
  Mux2 : Mux
  Mux3 : Mux
  Mux4 : Mux  Inputs=9
  Switch : Switch  Criteria=u2 ~= 0
  Switch1 : Switch  Criteria=u2 ~= 0
  Switch2 : Switch  Criteria=u2 ~= 0
  To File : ToFile  Filename=debud_vel_filters  MatrixName=debud_vel_filters
  disable1 : InportShadow
  disable2 : InportShadow
  sign convention{,1..3} (4 alike) : Gain  Gain=-1
  sw_conf{1..12} (12 alike) : InportShadow  Port=2
  dvarphi : Outport
  delta : Outport  Port=2
  ddelta : Outport  Port=3
  wires:
  SW1_sens/1 -> Bus Selector5/1
  SW2_sens/1 -> Bus Selector1/1
  [delta1] -> Mux1/1
  [delta2] -> Mux1/2
  [ddelta2] -> Mux2/2
  [ddelta1] -> Mux2/1
  SW3_sens/1 -> Bus Selector10/1
  [delta3] -> Mux1/3
  [ddelta3] -> Mux2/3
  SW4_sens/1 -> Bus Selector14/1
  [delta4] -> Mux1/4
  [ddelta4] -> Mux2/4
  Mux1/1 -> Add/2
  Mux3/1 -> Add/1
  Bus Selector4/1 -> Mux3/1  "<pivot_offs_sw1>"
  Bus Selector4/2 -> Mux3/2  "<pivot_offs_sw2>"
  Bus Selector4/3 -> Mux3/3  "<pivot_offs_sw3>"
  Bus Selector4/4 -> Mux3/4  "<pivot_offs_sw4>"
  Bus Selector5/3 -> Glitch removal + LP filter2/1(encoder)  "<encoder_pivot>"
  sign convention/1 -> Mux/2
  sign convention1/1 -> Mux/4
  sign convention2/1 -> Mux/6
  sign convention3/1 -> Mux/8
  Add/1 -> Switch/3
  Switch/1 -> delta/1
  disable/1 -> Switch/2
  Constant/1 -> Switch/1
  Switch1/1 -> ddelta/1
  Mux2/1 -> Switch1/3
  Constant1/1 -> Switch1/1
  disable1/1 -> Switch1/2
  disable2/1 -> Switch2/2
  Constant2/1 -> Switch2/1
  Mux/1 -> Switch2/3
  Switch2/1 -> dvarphi/1
  sw_conf/1 -> Bus Selector4/1
  sw_conf1/1 -> Bus Selector6/1
  sw_conf2/1 -> Bus Selector7/1
  sw_conf3/1 -> Bus Selector8/1
  sw_conf6/1 -> Bus Selector9/1
  sw_conf4/1 -> Bus Selector2/1
  sw_conf5/1 -> Bus Selector3/1
  sw_conf9/1 -> Bus Selector13/1
  sw_conf7/1 -> Bus Selector11/1
  sw_conf8/1 -> Bus Selector12/1
  sw_conf12/1 -> Bus Selector17/1
  sw_conf10/1 -> Bus Selector15/1
  sw_conf11/1 -> Bus Selector16/1
  [dvarphi1_1] -> Mux/1
  [dvarphi1_2] -> sign convention/1
  [dvarphi2_1] -> Mux/3
  [dvarphi2_2] -> sign convention1/1
  [dvarphi3_1] -> Mux/5
  [dvarphi3_2] -> sign convention2/1
  [dvarphi4_1] -> Mux/7
  [dvarphi4_2] -> sign convention3/1
  Mux4/1 -> To File/1
  Bus Selector5/1 -> Glitch removal + LP filter/1(encoder)  "<encoder_1>"
  Bus Selector6/1 -> Glitch removal + LP filter/2(LPF_fhz)  "<dvarphi_LPF_fhz>"
  Glitch removal + LP filter/1(out) -> [dvarphi1_1]
  Bus Selector7/1 -> Glitch removal + LP filter1/2(LPF_fhz)  "<dvarphi_LPF_fhz>"
  Bus Selector5/2 -> Glitch removal + LP filter1/1(encoder)  "<encoder_2>"
  Bus Selector8/1 -> Glitch removal + LP filter2/2(LPF_fhz)  "<ddelta_LPF_fhz>"
  Glitch removal + LP filter1/1(out) -> [dvarphi1_2]
  Glitch removal + LP filter2/1(encoder_out) -> [delta1]
  Glitch removal + LP filter2/2(vel_out) -> [ddelta1]
  Bus Selector2/1 -> Glitch removal + LP filter3/2(LPF_fhz)  "<dvarphi_LPF_fhz>"
  Bus Selector9/1 -> Glitch removal + LP filter5/2(LPF_fhz)  "<ddelta_LPF_fhz>"
  Bus Selector3/1 -> Glitch removal + LP filter4/2(LPF_fhz)  "<dvarphi_LPF_fhz>"
  Glitch removal + LP filter5/2(vel_out) -> [ddelta2]
  Glitch removal + LP filter3/1(out) -> [dvarphi2_1]
  Glitch removal + LP filter5/1(encoder_out) -> [delta2]
  Glitch removal + LP filter4/1(out) -> [dvarphi2_2]
  Bus Selector1/1 -> Glitch removal + LP filter3/1(encoder)  "<encoder_1>"
  Bus Selector1/2 -> Glitch removal + LP filter4/1(encoder)  "<encoder_2>"
  Bus Selector1/3 -> Glitch removal + LP filter5/1(encoder)  "<encoder_pivot>"
  Bus Selector13/1 -> Glitch removal + LP filter8/2(LPF_fhz)  "<ddelta_LPF_fhz>"
  Bus Selector10/1 -> Glitch removal + LP filter6/1(encoder)  "<encoder_1>"
  Glitch removal + LP filter7/1(out) -> [dvarphi3_2]
  Glitch removal + LP filter6/1(out) -> [dvarphi3_1]
  Bus Selector12/1 -> Glitch removal + LP filter7/2(LPF_fhz)  "<dvarphi_LPF_fhz>"
  Bus Selector10/3 -> Glitch removal + LP filter8/1(encoder)  "<encoder_pivot>"
  Glitch removal + LP filter8/1(encoder_out) -> [delta3]
  Glitch removal + LP filter8/2(vel_out) -> [ddelta3]
  Bus Selector11/1 -> Glitch removal + LP filter6/2(LPF_fhz)  "<dvarphi_LPF_fhz>"
  Bus Selector10/2 -> Glitch removal + LP filter7/1(encoder)  "<encoder_2>"
  Bus Selector17/1 -> Glitch removal + LP filter11/2(LPF_fhz)  "<ddelta_LPF_fhz>"
  Bus Selector14/1 -> Mux4/1, Glitch removal + LP filter9/1(encoder)  "<encoder_1>"
  Glitch removal + LP filter10/2(out) -> Mux4/6, [dvarphi4_2]
  Glitch removal + LP filter9/2(out) -> [dvarphi4_1], Mux4/3
  Bus Selector16/1 -> Glitch removal + LP filter10/2(LPF_fhz)  "<dvarphi_LPF_fhz>"
  Bus Selector14/3 -> Mux4/7, Glitch removal + LP filter11/1(encoder)  "<encoder_pivot>"
  Glitch removal + LP filter11/1(encoder_out) -> Mux4/8, [delta4]
  Glitch removal + LP filter11/2(vel_out) -> Mux4/9, [ddelta4]
  Bus Selector15/1 -> Glitch removal + LP filter9/2(LPF_fhz)  "<dvarphi_LPF_fhz>"
  Bus Selector14/2 -> Mux4/4, Glitch removal + LP filter10/1(encoder)  "<encoder_2>"
  Glitch removal + LP filter9/1(enc_out) -> Mux4/2
  Glitch removal + LP filter10/1(enc_out) -> Mux4/5

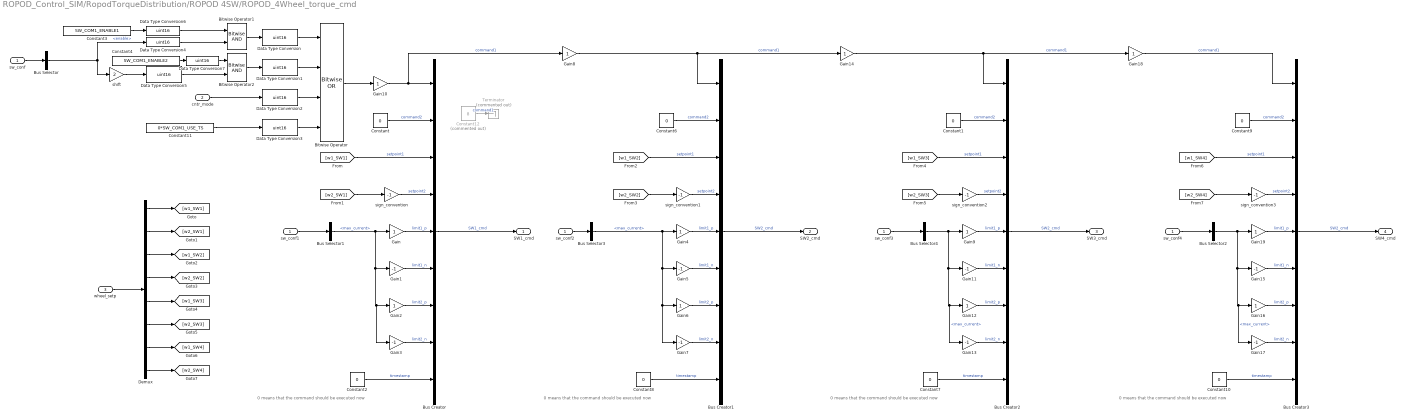
== system ROPOD_Control_SIM/RopodTorqueDistribution/ROPOD 4SW/ROPOD_4Wheel_torque_cmd ==
  note: 0 means that the command should be executed now
  note: 0 means that the command should be executed now
  note: 0 means that the command should be executed now
  note: 0 means that the command should be executed now
  sw_conf : Inport
  cntr_mode : Inport  Port=2
  wheel_setp : Inport  Port=3
  Bitwise Operator : simulink/Logic and Bit Operations/Bitwise Operator  logicop=OR  UseBitMask=off  NumInputPorts=4  BitMask=bin2dec('11011001')  BitMaskRealWorld=Stored Integer
  Bitwise Operator1 : simulink/Logic and Bit Operations/Bitwise Operator  logicop=AND  UseBitMask=off  NumInputPorts=2  BitMask=bin2dec('11011001')  BitMaskRealWorld=Stored Integer
  Bitwise Operator2 : simulink/Logic and Bit Operations/Bitwise Operator  logicop=AND  UseBitMask=off  NumInputPorts=2  BitMask=bin2dec('11011001')  BitMaskRealWorld=Stored Integer
  Bus Creator{,1..3} (4 alike) : BusCreator  Inputs=9
  Bus Selector : BusSelector  OutputSignals=enable
  Bus Selector{1..4} (4 alike) : BusSelector  OutputSignals=max_current
  Constant{,1..2,6..10} (8 alike) : Constant  Value=0
  Constant11 : Constant  Value=0*SW_COM1_USE_TS
  Constant12 : Constant  Commented=on  Value=8
  Constant3 : Constant  Value=SW_COM1_ENABLE1
  Constant4 : Constant  Value=SW_COM1_ENABLE2
  Data Type Conversion{,1..7} (8 alike) : DataTypeConversion  OutDataTypeStr=uint16
  Demux : Demux  Outputs=8
  Gain{,2,4,6,9,12,16,19} (8 alike) : Gain
  Gain{1,3,5,7,11,13,15,17} (8 alike) : Gain  Gain=-1
  Gain{8,10,14,18} (4 alike) : Gain  OutDataTypeStr=double
  Terminator : Terminator  Commented=on
  shift : Gain  Gain=2
  sign_convention{,1..3} (4 alike) : Gain  Gain=-1
  sw_conf{1..4} (4 alike) : InportShadow
  SW1_cmd : Outport
  SW2_cmd : Outport  Port=2
  SW3_cmd : Outport  Port=3
  SW4_cmd : Outport  Port=4
  wires:
  Bus Creator/1 -> SW1_cmd/1  "SW1_cmd"
  Constant2/1 -> Bus Creator/9  "timestamp"
  Constant/1 -> Bus Creator/2  "command2"
  [w1_SW1] -> Bus Creator/3  "setpoint1"
  Bus Selector1/1 -> Gain3/1, Gain2/1, Gain1/1, Gain/1  "<max_current>"
  [w2_SW1] -> sign_convention/1
  [w2_SW2] -> sign_convention1/1
  [w1_SW2] -> Bus Creator1/3  "setpoint1"
  Constant6/1 -> Bus Creator1/2  "command2"
  Constant8/1 -> Bus Creator1/9  "timestamp"
  Bus Creator1/1 -> SW2_cmd/1  "SW2_cmd"
  Demux/4 -> [w2_SW2]
  Demux/1 -> [w1_SW1]
  Demux/2 -> [w2_SW1]
  Demux/3 -> [w1_SW2]
  wheel_setp/1 -> Demux/1
  Gain/1 -> Bus Creator/5  "limit1_p"
  Gain1/1 -> Bus Creator/6  "limit1_n"
  Gain2/1 -> Bus Creator/7  "limit2_p"
  Gain3/1 -> Bus Creator/8  "limit2_n"
  Gain6/1 -> Bus Creator1/7  "limit2_p"
  Gain4/1 -> Bus Creator1/5  "limit1_p"
  Gain5/1 -> Bus Creator1/6  "limit1_n"
  Gain7/1 -> Bus Creator1/8  "limit2_n"
  Bus Selector3/1 -> Gain7/1, Gain6/1, Gain5/1, Gain4/1  "<max_current>"
  Gain8/1 -> Gain14/1, Bus Creator1/1  "command1"
  Bitwise Operator/1 -> Gain10/1
  Bitwise Operator1/1 -> Data Type Conversion/1
  Data Type Conversion2/1 -> Bitwise Operator/3
  Data Type Conversion1/1 -> Bitwise Operator/2
  Data Type Conversion3/1 -> Bitwise Operator/4
  Bitwise Operator2/1 -> Data Type Conversion1/1
  Data Type Conversion/1 -> Bitwise Operator/1
  Constant11/1 -> Data Type Conversion3/1
  sw_conf/1 -> Bus Selector/1
  Bus Selector/1 -> Data Type Conversion4/1, shift/1  "<enable>"
  sw_conf1/1 -> Bus Selector1/1
  Gain10/1 -> Bus Creator/1, Gain8/1  "command1"
  sw_conf2/1 -> Bus Selector3/1
  Gain12/1 -> Bus Creator2/7  "limit2_p"
  [w2_SW3] -> sign_convention2/1
  Bus Creator2/1 -> SW3_cmd/1  "SW2_cmd"
  Gain13/1 -> Bus Creator2/8  "limit2_n"
  sw_conf3/1 -> Bus Selector4/1
  Gain11/1 -> Bus Creator2/6  "limit1_n"
  Constant1/1 -> Bus Creator2/2  "command2"
  [w1_SW3] -> Bus Creator2/3  "setpoint1"
  Constant7/1 -> Bus Creator2/9  "timestamp"
  Bus Selector4/1 -> Gain13/1, Gain12/1, Gain11/1, Gain9/1  "<max_current>"
  Gain9/1 -> Bus Creator2/5  "limit1_p"
  Demux/5 -> [w1_SW3]
  Demux/6 -> [w2_SW3]
  Gain19/1 -> Bus Creator3/5  "limit1_p"
  Bus Selector2/1 -> Gain19/1, Gain15/1, Gain16/1, Gain17/1  "<max_current>"
  Constant10/1 -> Bus Creator3/9  "timestamp"
  [w1_SW4] -> Bus Creator3/3  "setpoint1"
  Constant9/1 -> Bus Creator3/2  "command2"
  Gain15/1 -> Bus Creator3/6  "limit1_n"
  sw_conf4/1 -> Bus Selector2/1
  Gain17/1 -> Bus Creator3/8  "limit2_n"
  Bus Creator3/1 -> SW4_cmd/1  "SW2_cmd"
  [w2_SW4] -> sign_convention3/1
  Gain16/1 -> Bus Creator3/7  "limit2_p"
  Gain18/1 -> Bus Creator3/1  "command1"
  Gain14/1 -> Gain18/1, Bus Creator2/1  "command1"
  Demux/7 -> [w1_SW4]
  Demux/8 -> [w2_SW4]
  shift/1 -> Data Type Conversion5/1
  Data Type Conversion4/1 -> Bitwise Operator1/2
  Data Type Conversion5/1 -> Bitwise Operator2/2
  Constant3/1 -> Data Type Conversion6/1
  Data Type Conversion6/1 -> Bitwise Operator1/1
  Constant4/1 -> Data Type Conversion7/1
  Data Type Conversion7/1 -> Bitwise Operator2/1
  sign_convention/1 -> Bus Creator/4  "setpoint2"
  sign_convention1/1 -> Bus Creator1/4  "setpoint2"
  sign_convention2/1 -> Bus Creator2/4  "setpoint2"
  sign_convention3/1 -> Bus Creator3/4  "setpoint2"
  Constant12/1 -> Terminator/1  "command1"
  cntr_mode/1 -> Data Type Conversion2/1

== system ROPOD_Control_SIM/RopodTorqueDistribution/ROPOD 4SW/empywheel ==
  SW4_cmd : Inport
  Bus Creator1 : BusCreator  Inputs=40
  Constant{,1..33,40..45} (40 alike) : Constant  Value=0
  Terminator : Terminator
  SW4_sens : Outport
  wires:
  SW4_cmd/1 -> Terminator/1
  Constant23/1 -> Bus Creator1/32  "imu_ts"
  Constant22/1 -> Bus Creator1/31  "voltage_bus"
  Constant7/1 -> Bus Creator1/8  "current_1_q"
  Constant31/1 -> Bus Creator1/26  "voltage_2_v"
  Constant32/1 -> Bus Creator1/33  "accel_x"
  Constant15/1 -> Bus Creator1/16  "temperature_1"
  Constant44/1 -> Bus Creator1/39  "temperature_imu"
  Constant9/1 -> Bus Creator1/10  "current_1_v"
  Constant21/1 -> Bus Creator1/30  "velocity_pivot"
  Constant45/1 -> Bus Creator1/40  "pressure"
  Constant10/1 -> Bus Creator1/11  "current_1_w"
  Constant16/1 -> Bus Creator1/17  "encoder_2"
  Constant3/1 -> Bus Creator1/4  "setpoint_ts"
  Constant28/1 -> Bus Creator1/23  "current_2_w"
  Constant41/1 -> Bus Creator1/36  "gyro_x"
  Constant4/1 -> Bus Creator1/5  "encoder_1"
  Constant6/1 -> Bus Creator1/7  "current_1_d"
  Constant18/1 -> Bus Creator1/27  "voltage_2_w"
  Constant12/1 -> Bus Creator1/13  "voltage_1_u"
  Constant43/1 -> Bus Creator1/38  "gyro_z"
  Constant25/1 -> Bus Creator1/20  "current_2_q"
  Constant42/1 -> Bus Creator1/37  "gyro_y"
  Constant19/1 -> Bus Creator1/28  "temperature_2"
  Constant8/1 -> Bus Creator1/9  "current_1_u"
  Constant14/1 -> Bus Creator1/15  "voltage_1_w"
  Constant29/1 -> Bus Creator1/24  "voltage_2"
  Constant30/1 -> Bus Creator1/25  "voltage_2_u"
  Constant27/1 -> Bus Creator1/22  "current_2_v"
  Constant/1 -> Bus Creator1/1  "status1"
  Constant1/1 -> Bus Creator1/2  "status2"
  Constant40/1 -> Bus Creator1/35  "accel_z"
  Constant11/1 -> Bus Creator1/12  "voltage_1"
  Constant5/1 -> Bus Creator1/6  "velocity_1"
  Constant13/1 -> Bus Creator1/14  "voltage_1_v"
  Constant24/1 -> Bus Creator1/19  "current_2_d"
  Constant17/1 -> Bus Creator1/18  "velocity_2"
  Constant20/1 -> Bus Creator1/29  "encoder_pivot"
  Constant33/1 -> Bus Creator1/34  "accel_y"
  Constant2/1 -> Bus Creator1/3  "sensor_ts"
  Constant26/1 -> Bus Creator1/21  "current_2_u"
  Bus Creator1/1 -> SW4_sens/1

== system ROPOD_Control_SIM/RopodTorqueDistribution/pivot damping cntr/Pivot controller ==
  dvarphi_error : Inport
  ena_w : Inport  Port=2
  platform_dvarphi_cntr_param : Inport  Port=3
  reset_int : Inport  Port=4
  Demux : Demux
  G_I_LL_LPF Controller1 : Subsystem
  G_I_LL_LPF Controller2 : Subsystem
  G_I_LL_LPF Controller3 : Subsystem
  G_I_LL_LPF Controller4 : Subsystem
  Gain{,6,8,10} (4 alike) : Gain  Gain=-1
  Gain{1,7,9,11} (4 alike) : Gain
  Mux : Mux  Inputs=8
  Product9 : Product
  varphi_tau_setp : Outport
  wires:
  Product9/1 -> Demux/1
  dvarphi_error/1 -> Product9/1
  [reset_int_cntr] -> G_I_LL_LPF Controller1/3(reset_integrator)
  Demux/1 -> G_I_LL_LPF Controller1/2(In)
  [param_dvarphi_cntr] -> G_I_LL_LPF Controller1/1(param)
  platform_dvarphi_cntr_param/1 -> [param_dvarphi_cntr]
  reset_int/1 -> [reset_int_cntr]
  [param_dvarphi_cntr] -> G_I_LL_LPF Controller2/1(param)
  [reset_int_cntr] -> G_I_LL_LPF Controller2/3(reset_integrator)
  Demux/2 -> G_I_LL_LPF Controller2/2(In)
  [reset_int_cntr] -> G_I_LL_LPF Controller4/3(reset_integrator)
  Demux/3 -> G_I_LL_LPF Controller3/2(In)
  Demux/4 -> G_I_LL_LPF Controller4/2(In)
  [param_dvarphi_cntr] -> G_I_LL_LPF Controller4/1(param)
  [param_dvarphi_cntr] -> G_I_LL_LPF Controller3/1(param)
  [reset_int_cntr] -> G_I_LL_LPF Controller3/3(reset_integrator)
  Mux/1 -> varphi_tau_setp/1
  ena_w/1 -> Product9/2
  G_I_LL_LPF Controller1/1(Out) -> Gain1/1, Gain/1
  G_I_LL_LPF Controller2/1(Out) -> Gain6/1, Gain7/1
  G_I_LL_LPF Controller3/1(Out) -> Gain9/1, Gain8/1
  G_I_LL_LPF Controller4/1(Out) -> Gain10/1, Gain11/1
  Gain/1 -> Mux/1
  Gain1/1 -> Mux/2
  Gain6/1 -> Mux/3
  Gain7/1 -> Mux/4
  Gain8/1 -> Mux/5
  Gain9/1 -> Mux/6
  Gain10/1 -> Mux/7
  Gain11/1 -> Mux/8
